simulink model "relative_DC_SK"  (R2021a)
settings: Solver=VariableStepAuto  StartTime=0.0  StopTime=time_sim*24  FixedStep=1  RelTol=1e-5
undefined symbols (not defined in the file or in its folder): e, init_conds, n, reference_conds, teta_0
libraries: pid_lib x2
settings Model: Creator=danie  LastModifiedBy=danie
settings SolverCC: AlgebraicLoopSolver=TrustRegion
settings DebuggingCC: SFMachineParentedDataDiag=warning

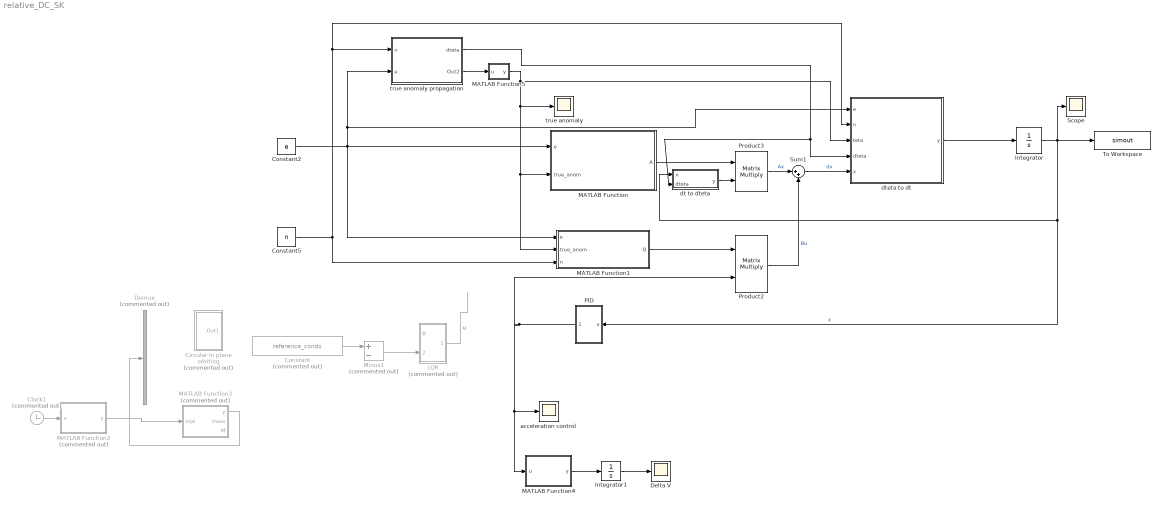
== system relative_DC_SK ==
  Circular in plane orbiting : Subsystem  Commented=on
  Clock1 : Clock  Commented=on
  Constant : Constant  Commented=on  Value=reference_conds
  Constant2 : Constant  Value=e
  Constant5 : Constant  Value=n
  Delta V : Scope
  Demux : Demux  Commented=on  Outputs=6
  Integrator : Integrator  InitialCondition=init_conds
  Integrator1 : Integrator
  LQR : Subsystem  Commented=on
  MATLAB Function : MATLAB Function  TreatAsAtomicUnit=on
  MATLAB Function1 : MATLAB Function  TreatAsAtomicUnit=on
  MATLAB Function2 : MATLAB Function  Commented=on  TreatAsAtomicUnit=on
  MATLAB Function3 : MATLAB Function  Commented=on  TreatAsAtomicUnit=on
  MATLAB Function4 : MATLAB Function  TreatAsAtomicUnit=on
  MATLAB Function5 : MATLAB Function  TreatAsAtomicUnit=on
  Minus1 : Sum  Commented=on  Inputs=+-
  PID : Subsystem
  Product2 : Product  SCDEnableBlockLinearizationSpecification=on  Multiplication=Matrix(*)
  Product3 : Product  SCDEnableBlockLinearizationSpecification=on  Multiplication=Matrix(*)
  Scope : Scope
  Sum1 : Sum  Inputs=|++
  To Workspace : ToWorkspace  VariableName=simout  SaveFormat=Timeseries  SampleTime=-1
  acceleration control : Scope
  dt to dteta : MATLAB Function  TreatAsAtomicUnit=on
  dteta to dt : MATLAB Function  TreatAsAtomicUnit=on
  true anomaly : Scope
  true anomaly propagation : Subsystem
  wires:
  Constant5/1 -> MATLAB Function1/3(n), true anomaly propagation/1(n), dteta to dt/2(n)
  MATLAB Function2/1(y) -> MATLAB Function3/1(mjd)
  MATLAB Function3/1(y) -> Demux/1
  Clock1/1 -> MATLAB Function2/1(u)
  MATLAB Function/1(A) -> Product3/1
  MATLAB Function1/1(B) -> Product2/1
  Integrator/1 -> Scope/1, To Workspace/1, PID/1(x), dt to dteta/1(x)  "x"
  Constant2/1 -> MATLAB Function1/1(e), MATLAB Function/1(e), true anomaly propagation/2(e), dteta to dt/1(e)
  LQR/1(Out1) -> ?  "u"
  Minus1/1 -> LQR/2(In2)
  Product3/1 -> Sum1/1  "Ax"
  Product2/1 -> Sum1/2  "Bu"
  Constant/1 -> Minus1/1
  Sum1/1 -> dteta to dt/5(x)  "dx"
  dteta to dt/1(y) -> Integrator/1
  dt to dteta/1(y) -> Product3/2
  true anomaly propagation/1(dteta) -> dteta to dt/4(dteta), dt to dteta/2(dteta)
  true anomaly propagation/2(Out2) -> MATLAB Function5/1(u)
  MATLAB Function5/1(y) -> MATLAB Function1/2(true_anom), MATLAB Function/2(true_anom), true anomaly/1, dteta to dt/3(teta)
  MATLAB Function4/1(y) -> Integrator1/1
  Integrator1/1 -> Delta V/1
  PID/1(Out1) -> MATLAB Function4/1(u), acceleration control/1, Product2/2

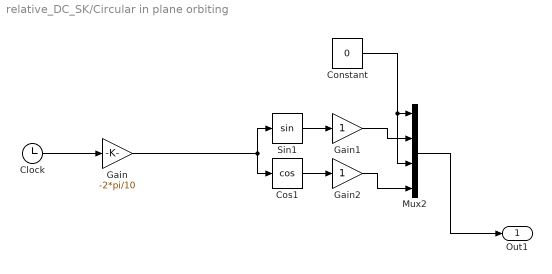
== system relative_DC_SK/Circular in plane orbiting ==
  Clock : Clock
  Constant : Constant  Value=0
  Cos1 : Trigonometry  Operator=cos
  Gain : Gain  Gain=-2*pi/10
  Gain1 : Gain
  Gain2 : Gain
  Mux2 : Mux
  Sin1 : Trigonometry
  Out1 : Outport
  wires:
  Gain/1 -> Cos1/1, Sin1/1
  Gain2/1 -> Mux2/4
  Clock/1 -> Gain/1
  Sin1/1 -> Gain1/1
  Cos1/1 -> Gain2/1
  Mux2/1 -> Out1/1
  Gain1/1 -> Mux2/2
  Constant/1 -> Mux2/3, Mux2/1

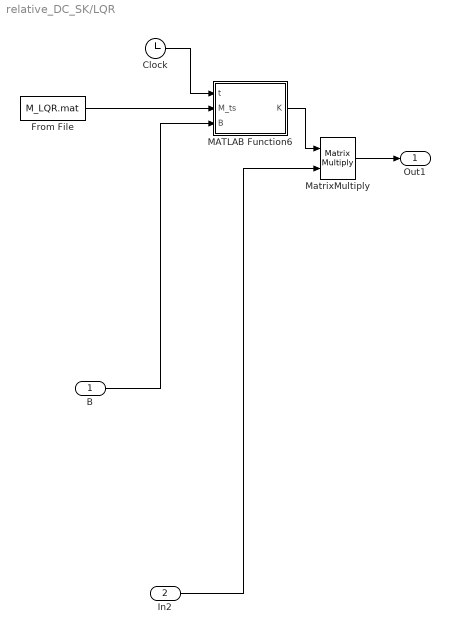
== system relative_DC_SK/LQR ==
  B : Inport
  In2 : Inport  Port=2
  Clock : Clock
  From File : FromFile  FileName=M_LQR.mat  SampleTime=0
  MATLAB Function6 : MATLAB Function  TreatAsAtomicUnit=on
  MatrixMultiply : Product  Multiplication=Matrix(*)
  Out1 : Outport
  wires:
  MATLAB Function6/1(K) -> MatrixMultiply/1
  From File/1 -> MATLAB Function6/2(M_ts)
  Clock/1 -> MATLAB Function6/1(t)
  MatrixMultiply/1 -> Out1/1
  B/1 -> MATLAB Function6/3(B)
  In2/1 -> MatrixMultiply/2

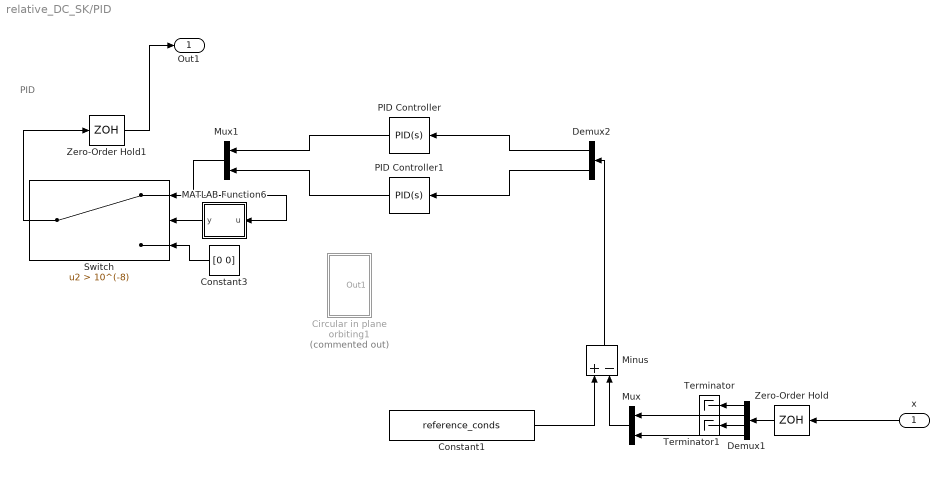
== system relative_DC_SK/PID ==
  note: PID
  x : Inport
  Circular in plane orbiting1 : Subsystem  Commented=on
  Constant1 : Constant  Value=reference_conds
  Constant3 : Constant  Value=[0 0]
  Demux1 : Demux
  Demux2 : Demux  Outputs=2
  MATLAB Function6 : MATLAB Function  TreatAsAtomicUnit=on
  Minus : Sum  Inputs=+-
  Mux : Mux  Inputs=2
  Mux1 : Mux  Inputs=2
  PID Controller : pid_lib/PID Controller  Controller=PID  Form=Parallel  TimeDomain=Continuous-time  UseExternalTs=off  SampleTime=-1  IntegratorMethod=Forward Euler  FilterMethod=Forward Euler  ControllerParametersSource=internal  P=7.92636168824504e-06  I=8.03590913043914e-10  D=0.0173713562043106  UseFilter=on  N=1.98600740388307  TunerSelectOption=Transfer Function Based (PID Tuner App)  InitialConditionSource=internal  InitialConditionForIntegrator=0  InitialConditionForFilter=0  DifferentiatorICPrevScaledInput=0  ExternalReset=none  TrackingMode=off  Kt=1  LimitOutput=off  SatLimitsSource=internal  UpperSaturationLimit=inf  LowerSaturationLimit=-inf  LinearizeAsGain=on  AntiWindupMode=none  Kb=1  POutMin=[]  POutMax=[]  IOutMin=[]  IOutMax=[]  DOutMin=[]  DOutMax=[]  NOutMin=[]  NOutMax=[]  SumOutMin=[]  SumOutMax=[]  SaturationOutMin=[]  SaturationOutMax=[]  PParamMin=[]  PParamMax=[]  IParamMin=[]  IParamMax=[]  DParamMin=[]  DParamMax=[]  NParamMin=[]  NParamMax=[]  KbParamMin=[]  KbParamMax=[]  KtParamMin=[]  KtParamMax=[]  KbOutMin=[]  KbOutMax=[]  KtOutMin=[]  KtOutMax=[]  IntegratorOutMin=[]  IntegratorOutMax=[]  FilterOutMin=[]  FilterOutMax=[]  SumI1OutMin=[]  SumI1OutMax=[]  SumI2OutMin=[]  SumI2OutMax=[]  SumI3OutMin=[]  SumI3OutMax=[]  SumI4OutMin=[]  SumI4OutMax=[]  SumDOutMin=[]  SumDOutMax=[]  DifferentiatorOutMin=[]  DifferentiatorOutMax=[]  FilterDiffOutCoefMin=[]  FilterDiffOutCoefMax=[]  ReciprocalOutMin=[]  ReciprocalOutMax=[]  SumDenOutMin=[]  SumDenOutMax=[]  SumNumOutMin=[]  SumNumOutMax=[]  DivideOutMin=[]  DivideOutMax=[]  UdiffTsProdOutMin=[]  UdiffTsProdOutMax=[]  NTsProdOutMin=[]  NTsProdOutMax=[]  UintegralTsProdOutMin=[]  UintegralTsProdOutMax=[]  UngainTsProdOutMin=[]  UngainTsProdOutMax=[]  IntegratorContinuousStateAttributes=''  IntegratorStateMustResolveToSignalObject=off  IntegratorRTWStateStorageClass=Auto  FilterContinuousStateAttributes=''  FilterStateMustResolveToSignalObject=off  FilterRTWStateStorageClass=Auto  ParallelPVariant=InternalParameters  IdealPVariant=Disabled  IVariant=InternalParameters  DVariant=InternalParameters  IntegratorVariant=Continuous  SatVariant=Disabled  AWVariant=Passthrough  PCopyVariant=Disabled  TRVariant=Disabled  FdbkBlocksVariant=Forward  IdealPFdbkVariant=Disabled  SatFdbkVariant=Disabled  DerivativeFilterVariant=ContFilter  NVariant=InternalParameters  NCopyVariant=Disabled  FilterICVariant=InternalICsFilter  IntegratorICVariant=InternalICs  ExternalResetVariant=Disabled  TRSumVariant=Passthrough  SumFdbkVariant=Disabled  SumVariant=Sum_PID  TsampFilterVariant=InternalTs  TsampNgainVariant=Passthrough  TsampIntegralVariant=Passthrough  ExternalSaturationOutDataTypeStr=Inherit: Same as second input
  PID Controller1 : pid_lib/PID Controller  Controller=PID  Form=Parallel  TimeDomain=Continuous-time  UseExternalTs=off  SampleTime=-1  IntegratorMethod=Forward Euler  FilterMethod=Forward Euler  ControllerParametersSource=internal  P=0.00250797878234495  I=1.46651362204143e-05  D=0.0971457531084103  UseFilter=on  N=0.212291335792304  TunerSelectOption=Transfer Function Based (PID Tuner App)  InitialConditionSource=internal  InitialConditionForIntegrator=0  InitialConditionForFilter=0  DifferentiatorICPrevScaledInput=0  ExternalReset=none  TrackingMode=off  Kt=1  LimitOutput=off  SatLimitsSource=internal  UpperSaturationLimit=inf  LowerSaturationLimit=-inf  LinearizeAsGain=on  AntiWindupMode=none  Kb=1  POutMin=[]  POutMax=[]  IOutMin=[]  IOutMax=[]  DOutMin=[]  DOutMax=[]  NOutMin=[]  NOutMax=[]  SumOutMin=[]  SumOutMax=[]  SaturationOutMin=[]  SaturationOutMax=[]  PParamMin=[]  PParamMax=[]  IParamMin=[]  IParamMax=[]  DParamMin=[]  DParamMax=[]  NParamMin=[]  NParamMax=[]  KbParamMin=[]  KbParamMax=[]  KtParamMin=[]  KtParamMax=[]  KbOutMin=[]  KbOutMax=[]  KtOutMin=[]  KtOutMax=[]  IntegratorOutMin=[]  IntegratorOutMax=[]  FilterOutMin=[]  FilterOutMax=[]  SumI1OutMin=[]  SumI1OutMax=[]  SumI2OutMin=[]  SumI2OutMax=[]  SumI3OutMin=[]  SumI3OutMax=[]  SumI4OutMin=[]  SumI4OutMax=[]  SumDOutMin=[]  SumDOutMax=[]  DifferentiatorOutMin=[]  DifferentiatorOutMax=[]  FilterDiffOutCoefMin=[]  FilterDiffOutCoefMax=[]  ReciprocalOutMin=[]  ReciprocalOutMax=[]  SumDenOutMin=[]  SumDenOutMax=[]  SumNumOutMin=[]  SumNumOutMax=[]  DivideOutMin=[]  DivideOutMax=[]  UdiffTsProdOutMin=[]  UdiffTsProdOutMax=[]  NTsProdOutMin=[]  NTsProdOutMax=[]  UintegralTsProdOutMin=[]  UintegralTsProdOutMax=[]  UngainTsProdOutMin=[]  UngainTsProdOutMax=[]  IntegratorContinuousStateAttributes=''  IntegratorStateMustResolveToSignalObject=off  IntegratorRTWStateStorageClass=Auto  FilterContinuousStateAttributes=''  FilterStateMustResolveToSignalObject=off  FilterRTWStateStorageClass=Auto  ParallelPVariant=InternalParameters  IdealPVariant=Disabled  IVariant=InternalParameters  DVariant=InternalParameters  IntegratorVariant=Continuous  SatVariant=Disabled  AWVariant=Passthrough  PCopyVariant=Disabled  TRVariant=Disabled  FdbkBlocksVariant=Forward  IdealPFdbkVariant=Disabled  SatFdbkVariant=Disabled  DerivativeFilterVariant=ContFilter  NVariant=InternalParameters  NCopyVariant=Disabled  FilterICVariant=InternalICsFilter  IntegratorICVariant=InternalICs  ExternalResetVariant=Disabled  TRSumVariant=Passthrough  SumFdbkVariant=Disabled  SumVariant=Sum_PID  TsampFilterVariant=InternalTs  TsampNgainVariant=Passthrough  TsampIntegralVariant=Passthrough  ExternalSaturationOutDataTypeStr=Inherit: Same as second input
  Switch : Switch  Criteria=u2 > Threshold  Threshold=10^(-8)
  Terminator : Terminator
  Terminator1 : Terminator
  Zero-Order Hold : ZeroOrderHold
  Zero-Order Hold1 : ZeroOrderHold
  Out1 : Outport
  wires:
  Minus/1 -> Demux2/1
  Zero-Order Hold/1 -> Demux1/1
  Demux1/2 -> Mux/1
  Constant1/1 -> Minus/1
  Demux2/2 -> PID Controller1/1
  PID Controller1/1 -> Mux1/2
  Mux/1 -> Minus/2
  MATLAB Function6/1(y) -> Switch/2
  Mux1/1 -> Switch/1, MATLAB Function6/1(u)
  Demux1/4 -> Mux/2
  Constant3/1 -> Switch/3
  Switch/1 -> Zero-Order Hold1/1
  Demux2/1 -> PID Controller/1
  PID Controller/1 -> Mux1/1
  x/1 -> Zero-Order Hold/1
  Zero-Order Hold1/1 -> Out1/1
  Demux1/1 -> Terminator/1
  Demux1/3 -> Terminator1/1

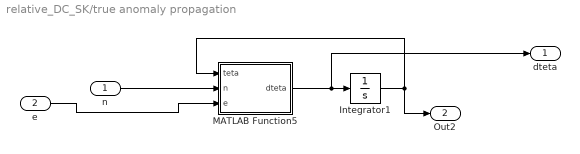
== system relative_DC_SK/true anomaly propagation ==
  n : Inport
  e : Inport  Port=2
  Integrator1 : Integrator  InitialCondition=teta_0
  MATLAB Function5 : MATLAB Function  TreatAsAtomicUnit=on
  dteta : Outport
  Out2 : Outport  Port=2
  wires:
  MATLAB Function5/1(dteta) -> dteta/1, Integrator1/1
  e/1 -> MATLAB Function5/3(e)
  Integrator1/1 -> Out2/1, MATLAB Function5/1(teta)
  n/1 -> MATLAB Function5/2(n)

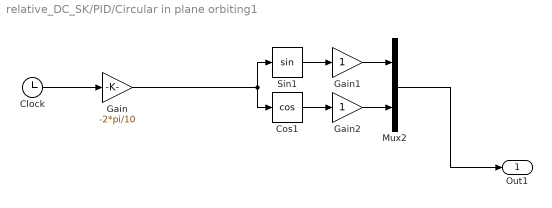
== system relative_DC_SK/PID/Circular in plane orbiting1 ==
  Clock : Clock
  Cos1 : Trigonometry  Operator=cos
  Gain : Gain  Gain=-2*pi/10
  Gain1 : Gain
  Gain2 : Gain
  Mux2 : Mux  Inputs=2
  Sin1 : Trigonometry
  Out1 : Outport
  wires:
  Gain/1 -> Cos1/1, Sin1/1
  Gain2/1 -> Mux2/2
  Clock/1 -> Gain/1
  Sin1/1 -> Gain1/1
  Cos1/1 -> Gain2/1
  Mux2/1 -> Out1/1
  Gain1/1 -> Mux2/1

== matlab function relative_DC_SK/MATLAB Function1 ==
  data: e input; B output; true_anom input; n input
function B = B_ss(e,true_anom,n)
B=((1-(e^2))^3)/(((1+e*cos(true_anom))^4)*(n^2))*[1 0; 0 0; 0 1; 0 0];

== matlab function relative_DC_SK/MATLAB Function ==
  data: e input; A output; true_anom input
function A = A_ss(e,true_anom)
A=[ 2*e*sin(true_anom)/(1+e*cos(true_anom)), (3+e*cos(true_anom))/(1+e*cos(true_anom)), 2, -2*e*sin(true_anom)/(1+e*cos(true_anom)); 
    1, 0, 0, 0;
   -2, 2*e*sin(true_anom)/(1+e*cos(true_anom)), 2*e*sin(true_anom)/(1+e*cos(true_anom)), e*cos(true_anom)/(1+e*cos(true_anom));
   0, 0, 1, 0];

== matlab function relative_DC_SK/MATLAB Function2 ==
  data: u input; y output
function y = time_conv(u)
y=double(60676+((u/3600)/24));

== matlab function relative_DC_SK/MATLAB Function3 ==
  data: mjd input; y output; mass output; M output
function [y, mass, M]= get_eph(mjd)
    [y, mass, M]=ephNEO(mjd,28);

== matlab function relative_DC_SK/PID/MATLAB Function6 ==
  data: u input; y output
function y = fcn(u)

y = norm(u);

== matlab function relative_DC_SK/MATLAB Function4 ==
  data: u input; y output
function y = fcn(u)

y =norm(u);

== matlab function relative_DC_SK/LQR/MATLAB Function6 ==
  data: t input; M_ts input; K output; B input
function K = fcn(t,M_ts,B)
flag=0;
% for i=1:(length(M_ts.Time)-1)
%     if and(t>=M_ts.Time(i),t<M_ts.Time(i+1))
%         M=M_ts.data(i);
%         flag=1;
%         break
%     else
%         M=zeros(4,4)
%     end
% end
M=reshape(M_ts,4,4);
K=-B.'*M;

== matlab function relative_DC_SK/true anomaly propagation/MATLAB Function5 ==
  data: teta input; n input; dteta output; e input
function dteta = fcn(teta,n,e)
dteta=(n*(1+e*cos(teta))^2)/((1-e^2)^1.5);

== matlab function relative_DC_SK/dteta to dt ==
  data: e input; y output; n input; teta input; dteta input; x input
function y = fcn(e,n,teta,dteta,x)
y=x;
y(1)=x(1)*(dteta^2)+dteta*(-(n*2*(1+e*cos(teta))*e*sin(teta)/((1-e^2)^1.5)))*x(2);
y(2)=x(2)*dteta;
y(3)=x(3)*(dteta^2)+dteta*(-(n*2*(1+e*cos(teta))*e*sin(teta)/((1-e^2)^1.5)))*x(4);
y(4)=x(4)*dteta;

== matlab function relative_DC_SK/dt to dteta ==
  data: x input; y output; dteta input
function y = fcn(x,dteta)
y=x;
y(1)=x(1)/dteta;
y(3)=x(3)/dteta;

== matlab function relative_DC_SK/MATLAB Function5 ==
  data: u input; y output
function y = fcn(u)

y = mod(u,2*pi);
